simulink model "dc_motor"  (R2019b)
settings: Solver=VariableStepAuto  StartTime=0.0  StopTime=100  RelTol=1e-3
model workspace: external: MATLAB File D:\Personal Projects\ELEC-391\Mini-Project\constants.m (data not in the file)
values from neighbouring files (symbols this model uses):
  K_b = 16.11    [constants.m]
  K_m = 0.062    [constants.m]
  Ze_den = [.002 1.0]    [constants.m]
  Ze_num = [1]    [constants.m]
  Zm_den = [0.00013 0.0000102]    [constants.m]
  Zm_num = [1]    [constants.m]
settings Model: OrderedModelArguments=off  Creator=matti  LastModifiedBy=matti

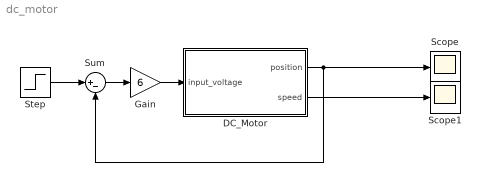
== system dc_motor ==
  "DC_Motor " : Subsystem
  Gain : Gain  Gain=6
  Scope : Scope
  Scope1 : Scope
  Step : Step  After=3.14  SampleTime=0
  Sum : Sum  Inputs=|+-
  wires:
  "DC_Motor "/1(position) -> Scope/1, Sum/2
  "DC_Motor "/2(speed) -> Scope1/1
  Gain/1 -> "DC_Motor "/1(input_voltage)
  Sum/1 -> Gain/1
  Step/1 -> Sum/1

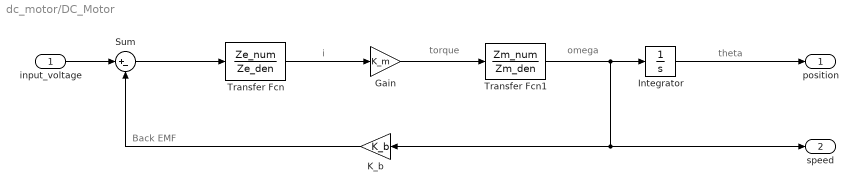
== system dc_motor/DC_Motor  ==
  note: theta
  note: omega
  note: torque
  note: i
  note: Back EMF
  input_voltage : Inport
  Gain : Gain  Gain=K_m
  Integrator : Integrator
  K_b : Gain  Gain=K_b
  Sum : Sum  Inputs=|+-
  Transfer Fcn : TransferFcn  Numerator=Ze_num  Denominator=Ze_den
  Transfer Fcn1 : TransferFcn  Numerator=Zm_num  Denominator=Zm_den
  position : Outport
  speed : Outport  Port=2
  wires:
  Transfer Fcn1/1 -> speed/1, K_b/1, Integrator/1
  K_b/1 -> Sum/2
  Integrator/1 -> position/1
  Transfer Fcn/1 -> Gain/1
  Gain/1 -> Transfer Fcn1/1
  Sum/1 -> Transfer Fcn/1
  input_voltage/1 -> Sum/1
